simulink model "model_with_library_links"  (R2015b)
settings: Solver=ode4  StartTime=0.0  StopTime=1  FixedStep=50E-6  RelTol=1e-3
undefined symbols (not defined in the file): param_198a5ba83d87bd2227ff7bec4eafe564
libraries: library x1
settings Model: Creator=Wippenbeck  LastModifiedBy=bertram
settings DataIOCC: SaveFormat=Array  ReturnWorkspaceOutputs=on  SignalLoggingName=STOVICAL_LoggedSignals  ReturnWorkspaceOutputsName=simout_obj
settings DebuggingCC: SolverPrmCheckMsg=warning
settings HardwareCC: ProdBitPerPointer=32  ProdLargestAtomicFloat=None  ProdIntDivRoundTo=Undefined  ProdEndianess=Unspecified  ProdWordSize=32  ProdHWDeviceType=32-bit Generic
settings GRTTargetCC: GeneratePreprocessorConditionals=Disable all
settings ConfigComp: CovModelRefEnable=Off  CovSFcnEnable=off

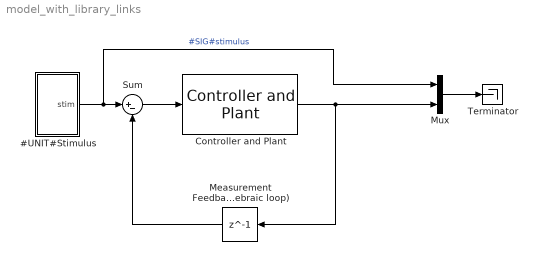
== system model_with_library_links ==
  #UNIT#Stimulus : Subsystem
  Controller and Plant : library/Controller and Plant
  Measurement Feedback (avoids algebraic loop) : Delay  DelayLength=1  InitialCondition=0
  Mux : Mux  Inputs=2
  Sum : Sum  Inputs=|+-
  Terminator : Terminator
  wires:
  Mux/1 -> Terminator/1
  #UNIT#Stimulus/1(stim) -> Sum/1, Mux/1  "#SIG#stimulus"
  Controller and Plant/1 -> Measurement Feedback (avoids algebraic loop)/1, Mux/2
  Measurement Feedback (avoids algebraic loop)/1 -> Sum/2
  Sum/1 -> Controller and Plant/1

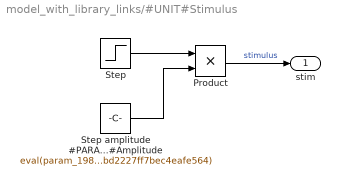
== system model_with_library_links/#UNIT#Stimulus ==
  Product : Product
  Step : Step  Time=0.1  SampleTime=0
  Step amplitude #PARAM#Amplitude : Constant  Value=eval(param_198a5ba83d87bd2227ff7bec4eafe564)
  stim : Outport
  wires:
  Step amplitude #PARAM#Amplitude/1 -> Product/2
  Product/1 -> stim/1  "stimulus"
  Step/1 -> Product/1
